simulink model "multiplexer"  (R2021a)
settings: Solver=VariableStepAuto  StartTime=0.0  StopTime=8  RelTol=1e-3
libraries: simulink x5
settings Model: Creator=hritw  LastModifiedBy=hritw

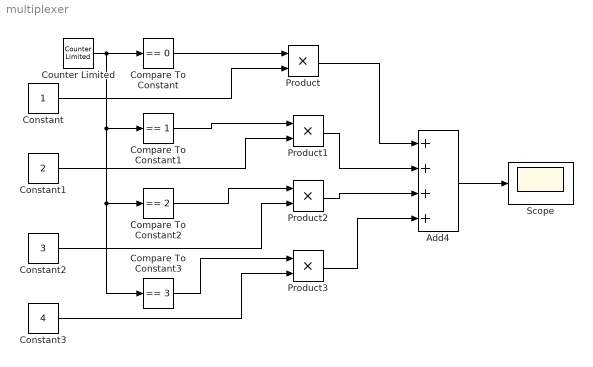
== system multiplexer ==
  Add4 : Sum  Inputs=++++
  Compare To Constant : simulink/Logic and Bit Operations/Compare To Constant  relop===  const=0  OutDataTypeStr=boolean
  Compare To Constant1 : simulink/Logic and Bit Operations/Compare To Constant  relop===  const=1  OutDataTypeStr=boolean
  Compare To Constant2 : simulink/Logic and Bit Operations/Compare To Constant  relop===  const=2  OutDataTypeStr=boolean
  Compare To Constant3 : simulink/Logic and Bit Operations/Compare To Constant  relop===  const=3  OutDataTypeStr=boolean
  Constant : Constant
  Constant1 : Constant  Value=2
  Constant2 : Constant  Value=3
  Constant3 : Constant  Value=4
  Counter Limited : simulink/Sources/Counter Limited  uplimit=4  tsamp=-1
  Product{,1..3} (4 alike) : Product
  Scope : Scope
  wires:
  Compare To Constant/1 -> Product/1
  Compare To Constant1/1 -> Product1/1
  Constant1/1 -> Product1/2
  Compare To Constant2/1 -> Product2/1
  Constant2/1 -> Product2/2
  Constant3/1 -> Product3/2
  Product/1 -> Add4/1
  Product1/1 -> Add4/2
  Product2/1 -> Add4/3
  Product3/1 -> Add4/4
  Add4/1 -> Scope/1
  Counter Limited/1 -> Compare To Constant3/1, Compare To Constant2/1, Compare To Constant1/1, Compare To Constant/1
  Compare To Constant3/1 -> Product3/1
  Constant/1 -> Product/2
